simulink library "pathFollowingCtrlAoATurbCoef_cl"  (R2022a)
settings: Solver=VariableStepAuto  StartTime=0.0  StopTime=10.0  RelTol=1e-3
undefined symbols (not defined in the file or in its folder): env, FLIGHTCONTROLLER, initializeBussesFromBlock, pthCtrl1, vhcl
libraries: slpidlib x5, velocityAngle_ul x2, pathFollowingCtrlAoATurb_cl x1, courseFollowLookAhead_cl x1, ctrlAllocMatrix3CompCoef_cl x1, eulAng2RotMat_ul x1, angleBtw2Vecs_ul x1, vrlib x1, alphaBeta_ul x1, gnd2TanRotation_ul x1, rotorTorqueCtrlDiscrete x1
settings Model: Creator=jldanie5  LastModifiedBy=jbfine
settings SolverCC: AlgebraicLoopSolver=TrustRegion
settings DataIOCC: ReturnWorkspaceOutputs=off
settings DebuggingCC: UnconnectedInputMsg=warning  UnconnectedOutputMsg=warning  UnconnectedLineMsg=warning  SFMachineParentedDataDiag=warning  ArithmeticOperatorsInVariantConditions=warning
settings SFSimCC: CustomCodeUndefinedFunction=UseInterfaceOnly

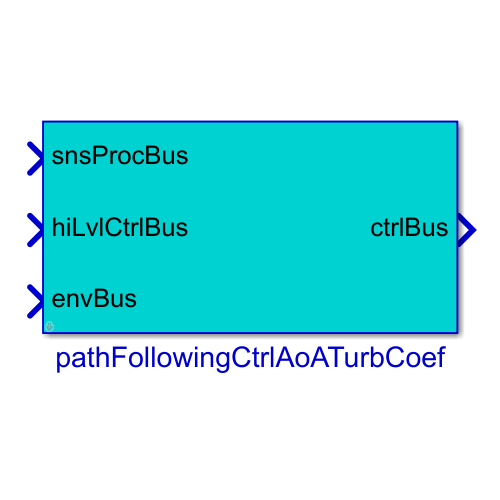
[thumbnail: Simulink's stored preview of the top-level diagram]
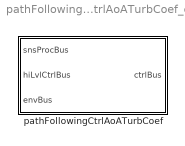
== system pathFollowingCtrlAoATurbCoef_cl ==
  pathFollowingCtrlAoATurbCoef : Subsystem  LoadFcn=initializeBussesFromBlock(gcb)  InitFcn=initializeBussesFromBlock(gcb)  StartFcn=initializeBussesFromBlock(gcb)  VariantControl=strcmpi(FLIGHTCONTROLLER,'pathFollowingControllerManta')  mask{initPosForInitSStar=vhcl.initPosVecGnd.Value, fluidDensity=env.water.density.Value, pathCtrl=pthCtrl1, aeroStruct=vhcl.struct('OCT.aeroSurf')}
      mask prompts: initPosForInitSStar "Initial Position"; fluidDensity "Fluid Density"; pathCtrl "Controller"; aeroStruct "Aerodynamic Structure"
      settings: MinAlgLoopOccurrences=on
      mask DialogControl Container3 Prompt: courseFollow Params
      mask DialogControl Container4 Prompt: setpointToOutput Params

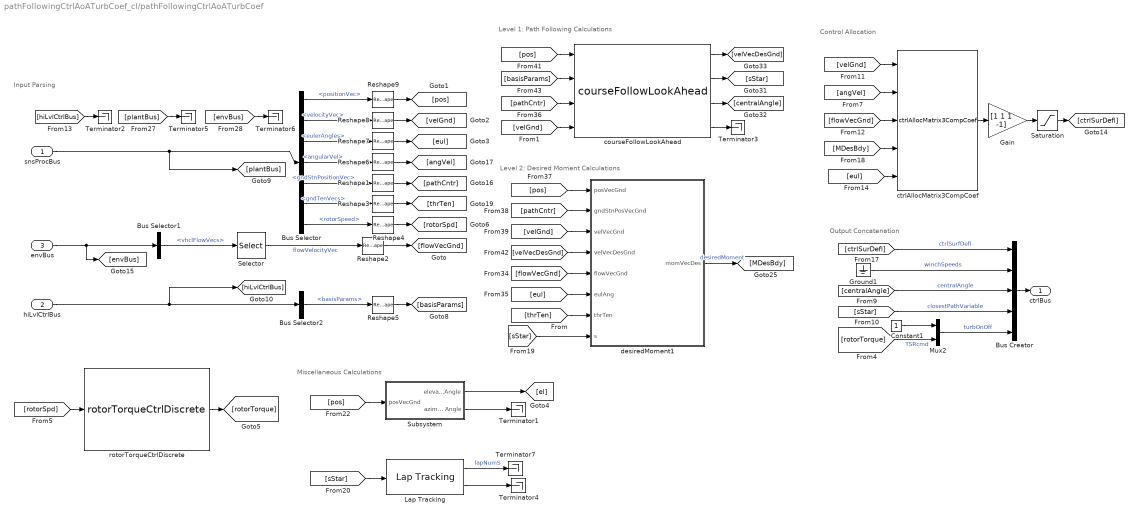
== system pathFollowingCtrlAoATurbCoef_cl/pathFollowingCtrlAoATurbCoef ==
  note: Control Allocation
  note: Miscellaneous Calculations
  note: Output Concatenation
  note: Input Parsing
  note: Level 1: Path Following Calculations
  note: Level 2: Desired Moment Calculations
  snsProcBus : Inport  OutDataTypeStr=Bus: sensorsProcessingBus
  hiLvlCtrlBus : Inport  Port=2
  envBus : Inport  Port=3  OutDataTypeStr=Bus: envBus
  Bus Creator : BusCreator  Inputs=5
  Bus Selector : BusSelector  OutputSignals=positionVec,velocityVec,eulerAngles,angularVel,gndStnPositionVec,gndTenVecs,rotorSpeed
  Bus Selector1 : BusSelector  OutputSignals=vhclFlowVecs
  Bus Selector2 : BusSelector  OutputSignals=basisParams
  Constant1 : Constant
  Gain : Gain  Gain=[1 1 1 -1]
  Ground1 : Ground
  Lap Tracking : pathFollowingCtrlAoATurb_cl/pathFollowingCtrlAoATurb/Lap Tracking  SystemSampleTime=-1  VariantActivationTime=update diagram  Latency=0  AutoFrameSizeCalculation=off
  Mux2 : Mux  Inputs=2
  Reshape{1..9} (9 alike) : Reshape  OutputDimensionality=Column vector (2-D)
  Saturation : Saturate  UpperLimit=30  LowerLimit=-30
  Selector : Selector  NumberOfDimensions=2  InputPortWidth=3  IndexOptions=Select all,Index vector (dialog)  Indices=[1 3],5  OutputSizes=1,1
  Subsystem : Subsystem
  Terminator{1..7} (7 alike) : Terminator
  courseFollowLookAhead : courseFollowLookAhead_cl/courseFollowLookAhead  SystemSampleTime=-1  VariantActivationTime=update diagram  Latency=0  AutoFrameSizeCalculation=off
  ctrlAllocMatrix3CompCoef : ctrlAllocMatrix3CompCoef_cl/ctrlAllocMatrix3CompCoef  aeroStruct=vhcl.struct('OCT.aeroSurf')  fluidDensity=fluidDensity  arms=vhcl.struct('OCT.thrAttch')
  desiredMoment1 : Subsystem
  rotorTorqueCtrlDiscrete : rotorTorqueCtrlDiscrete/rotorTorqueCtrlDiscrete  turb_struct=vhcl.struct('OCT.turb')  rho=rho
  ctrlBus : Outport  OutDataTypeStr=Bus: fltCtrlBus  VectorParamsAs1DForOutWhenUnconnected=off
  wires:
  Bus Selector/6 -> Reshape3/1  "<gndTenVecs>"
  Reshape3/1 -> [thrTen]
  snsProcBus/1 -> [plantBus], Bus Selector/1
  Bus Selector/2 -> Reshape8/1  "<velocityVec>"
  Bus Selector/1 -> Reshape9/1  "<positionVec>"
  Bus Selector/3 -> Reshape7/1  "<eulerAngles>"
  Bus Creator/1 -> ctrlBus/1
  Ground1/1 -> Bus Creator/2  "winchSpeeds"
  hiLvlCtrlBus/1 -> [hiLvlCtrlBus], Bus Selector2/1
  [centralAngle] -> Bus Creator/3  "centralAngle"
  [sStar] -> Bus Creator/4  "closestPathVariable"
  Bus Selector/4 -> Reshape6/1  "<angularVel>"
  [angVel] -> ctrlAllocMatrix3CompCoef/2
  [velGnd] -> ctrlAllocMatrix3CompCoef/1
  [flowVecGnd] -> ctrlAllocMatrix3CompCoef/3
  [MDesBdy] -> ctrlAllocMatrix3CompCoef/4
  [ctrlSurDefl] -> Bus Creator/1  "ctrlSurfDefl"
  Bus Selector2/1 -> Reshape5/1  "<basisParams>"
  Reshape5/1 -> [basisParams]
  Reshape2/1 -> [flowVecGnd]
  Reshape6/1 -> [angVel]
  Reshape7/1 -> [eul]
  Reshape8/1 -> [velGnd]
  Reshape9/1 -> [pos]
  [eul] -> ctrlAllocMatrix3CompCoef/5
  Selector/1 -> Reshape2/1  "flowVelocityVec"
  envBus/1 -> [envBus], Bus Selector1/1
  Bus Selector1/1 -> Selector/1  "<vhclFlowVecs>"
  Reshape1/1 -> [pathCntr]
  Bus Selector/5 -> Reshape1/1  "<gndStnPositionVec>"
  [pos] -> Subsystem/1(posVecGnd)
  Subsystem/2(azimuth Angle) -> Terminator1/1
  [plantBus] -> Terminator5/1
  [envBus] -> Terminator6/1
  [hiLvlCtrlBus] -> Terminator2/1
  Mux2/1 -> Bus Creator/5  "turbOnOff"
  Constant1/1 -> Mux2/1
  [rotorTorque] -> Mux2/2  "TSRcmd"
  [velVecDesGnd] -> desiredMoment1/4(velVecDesGnd)
  [velGnd] -> desiredMoment1/3(velVecGnd)
  [eul] -> desiredMoment1/6(eulAng)
  [basisParams] -> courseFollowLookAhead/2
  [pathCntr] -> desiredMoment1/2(gndStnPosVecGnd)
  courseFollowLookAhead/2 -> [sStar]
  [pos] -> desiredMoment1/1(posVecGnd)
  [pathCntr] -> courseFollowLookAhead/3
  desiredMoment1/1(momVecDes) -> [MDesBdy]  "desiredMoment"
  [pos] -> courseFollowLookAhead/1
  courseFollowLookAhead/3 -> [centralAngle]
  courseFollowLookAhead/4 -> Terminator3/1
  courseFollowLookAhead/1 -> [velVecDesGnd]
  [flowVecGnd] -> desiredMoment1/5(flowVecGnd)
  [thrTen] -> desiredMoment1/7(thrTen)
  [velGnd] -> courseFollowLookAhead/4
  Saturation/1 -> [ctrlSurDefl]
  [sStar] -> desiredMoment1/8(s)
  [rotorSpd] -> rotorTorqueCtrlDiscrete/1
  Reshape4/1 -> [rotorSpd]
  Bus Selector/7 -> Reshape4/1  "<rotorSpeed>"
  Subsystem/1(elevationAngle) -> [el]
  rotorTorqueCtrlDiscrete/1 -> [rotorTorque]
  ctrlAllocMatrix3CompCoef/1 -> Gain/1
  Gain/1 -> Saturation/1
  Lap Tracking/2 -> Terminator4/1
  Lap Tracking/1 -> Terminator7/1  "lapNumS"
  [sStar] -> Lap Tracking/1

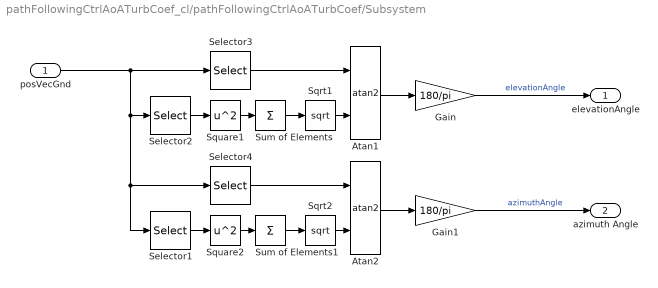
== system pathFollowingCtrlAoATurbCoef_cl/pathFollowingCtrlAoATurbCoef/Subsystem ==
  posVecGnd : Inport
  Atan1 : Trigonometry  Operator=atan2
  Atan2 : Trigonometry  Operator=atan2
  Gain : Gain  Gain=180/pi
  Gain1 : Gain  Gain=180/pi
  Selector1 : Selector  InputPortWidth=3  IndexOptions=Index vector (dialog)  Indices=1  OutputSizes=1
  Selector2 : Selector  InputPortWidth=3  IndexOptions=Index vector (dialog)  Indices=[1 2]  OutputSizes=1
  Selector3 : Selector  InputPortWidth=3  IndexOptions=Index vector (dialog)  Indices=3  OutputSizes=1
  Selector4 : Selector  InputPortWidth=3  IndexOptions=Index vector (dialog)  Indices=2  OutputSizes=1
  Sqrt1 : Sqrt
  Sqrt2 : Sqrt
  Square1 : Math  Operator=square  SignedPower=on
  Square2 : Math  Operator=square  SignedPower=on
  Sum of Elements : Sum  Inputs=+
  Sum of Elements1 : Sum  Inputs=+
  elevationAngle : Outport
  azimuth Angle : Outport  Port=2
  wires:
  Sqrt1/1 -> Atan1/2
  Square1/1 -> Sum of Elements/1
  Selector3/1 -> Atan1/1
  Sum of Elements/1 -> Sqrt1/1
  Atan1/1 -> Gain/1
  Selector2/1 -> Square1/1
  Gain/1 -> elevationAngle/1  "elevationAngle"
  Atan2/1 -> Gain1/1
  Square2/1 -> Sum of Elements1/1
  Sum of Elements1/1 -> Sqrt2/1
  Selector1/1 -> Square2/1
  posVecGnd/1 -> Selector1/1, Selector4/1, Selector2/1, Selector3/1
  Sqrt2/1 -> Atan2/2
  Selector4/1 -> Atan2/1
  Gain1/1 -> azimuth Angle/1  "azimuthAngle"

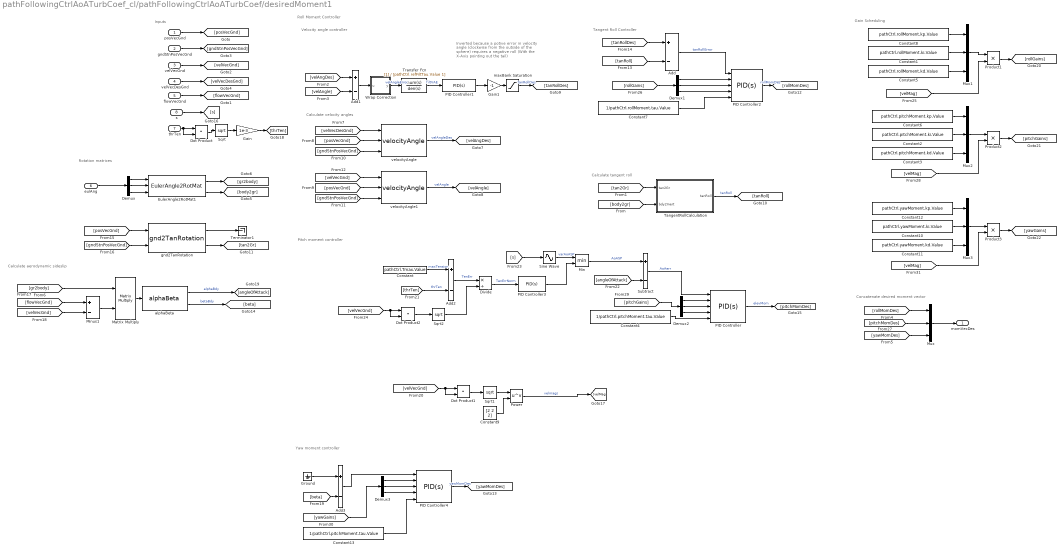
== system pathFollowingCtrlAoATurbCoef_cl/pathFollowingCtrlAoATurbCoef/desiredMoment1 ==
  note: Gain Scheduling
  note: Roll Moment Controller
  note: Calculate aerodynamic sideslip
  note: Concatenate desired moment vector
  note: Tangent Roll Controller
  note: Calculate tangent roll
  note: Calculate velocity angles
  note: Rotation matrices
  note: Inputs
  note: Velocity angle controller
  note: Inverted because a potive error
      | in velocity angle (clockwise from the
      | outside of the sphere) requires a negative
      | roll (With the X-Axis pointing out the tail)
  note: Pitch moment controller
  note: Yaw moment controller
  posVecGnd : Inport
  gndStnPosVecGnd : Inport  Port=2
  velVecGnd : Inport  Port=3
  velVecDesGnd : Inport  Port=4
  flowVecGnd : Inport  Port=5
  eulAng : Inport  Port=6
  thrTen : Inport  Port=7
  s : Inport  Port=8
  Add{,1..3} (4 alike) : Sum  Inputs=+-
  Constant : Constant  Value=pathCtrl.Tmax.Value
  Constant1 : Constant  Value=pathCtrl.rollMoment.ki.Value
  Constant10 : Constant  Value=pathCtrl.yawMoment.ki.Value
  Constant11 : Constant  Value=pathCtrl.yawMoment.kd.Value
  Constant12 : Constant  Value=pathCtrl.yawMoment.kp.Value
  Constant13 : Constant  Value=1/pathCtrl.pitchMoment.tau.Value
  Constant2 : Constant  Value=pathCtrl.pitchMoment.ki.Value
  Constant3 : Constant  Value=pathCtrl.pitchMoment.kd.Value
  Constant4 : Constant  Value=1/pathCtrl.pitchMoment.tau.Value
  Constant5 : Constant  Value=pathCtrl.rollMoment.kd.Value
  Constant6 : Constant  Value=pathCtrl.pitchMoment.kp.Value
  Constant7 : Constant  Value=1/pathCtrl.rollMoment.tau.Value
  Constant8 : Constant  Value=pathCtrl.rollMoment.kp.Value
  Constant9 : Constant  Value=[2 2 2]
  Demux{,1..3} (4 alike) : Demux  Outputs=3
  Divide : Product  Inputs=*/
  Dot Product : DotProduct  OutDataTypeStr=Inherit: Inherit via internal rule
  Dot Product1 : DotProduct  OutDataTypeStr=Inherit: Inherit via internal rule
  Dot Product2 : DotProduct  OutDataTypeStr=Inherit: Inherit via internal rule
  EulerAngle2RotMat1 : eulAng2RotMat_ul/EulerAngle2RotMat  SystemSampleTime=-1  VariantActivationTime=update diagram  Latency=0  AutoFrameSizeCalculation=off
  Gain : Gain  Gain=1e-3
  Gain1 : Gain  Gain=-1
  Ground : Ground
  Matrix Multiply : Product  Multiplication=Matrix(*)
  Min : MinMax  Inputs=2
  Minus1 : Sum  Inputs=+-
  Mux{,1..3} (4 alike) : Mux  Inputs=3
  PID Controller : slpidlib/PID Controller  Controller=PID  Form=Parallel  TimeDomain=Continuous-time  UseExternalTs=off  SampleTime=-1  IntegratorMethod=Forward Euler  FilterMethod=Forward Euler  ControllerParametersSource=external  P=pathCtrl.pitchMoment.kp.Value  I=pathCtrl.pitchMoment.ki.Value  UseKiTs=off  D=pathCtrl.pitchMoment.kd.Value  N=1/pathCtrl.pitchMoment.tau.Value  UseFilter=on  TunerSelectOption=Transfer Function Based (PID Tuner App)  InitialConditionSource=internal  InitialConditionForIntegrator=0  InitialConditionForFilter=0  DifferentiatorICPrevScaledInput=0  ExternalReset=none  TrackingMode=off  Kt=1  LimitOutput=off  SatLimitsSource=internal  UpperSaturationLimit=inf  LowerSaturationLimit=-100  LinearizeAsGain=on  AntiWindupMode=clamping  Kb=1  POutMin=[]  POutMax=[]  IOutMin=[]  IOutMax=[]  DOutMin=[]  DOutMax=[]  NOutMin=[]  NOutMax=[]  SumOutMin=[]  SumOutMax=[]  SaturationOutMin=[]  SaturationOutMax=[]  PParamMin=[]  PParamMax=[]  IParamMin=[]  IParamMax=[]  DParamMin=[]  DParamMax=[]  NParamMin=[]  NParamMax=[]  KbParamMin=[]  KbParamMax=[]  KtParamMin=[]  KtParamMax=[]  KbOutMin=[]  KbOutMax=[]  KtOutMin=[]  KtOutMax=[]  IntegratorOutMin=[]  IntegratorOutMax=[]  FilterOutMin=[]  FilterOutMax=[]  SumI1OutMin=[]  SumI1OutMax=[]  SumI2OutMin=[]  SumI2OutMax=[]  SumI3OutMin=[]  SumI3OutMax=[]  SumI4OutMin=[]  SumI4OutMax=[]  SumDOutMin=[]  SumDOutMax=[]  DifferentiatorOutMin=[]  DifferentiatorOutMax=[]  FilterDiffOutCoefMin=[]  FilterDiffOutCoefMax=[]  ReciprocalOutMin=[]  ReciprocalOutMax=[]  SumDenOutMin=[]  SumDenOutMax=[]  SumNumOutMin=[]  SumNumOutMax=[]  DivideOutMin=[]  DivideOutMax=[]  UdiffTsProdOutMin=[]  UdiffTsProdOutMax=[]  NTsProdOutMin=[]  NTsProdOutMax=[]  UintegralTsProdOutMin=[]  UintegralTsProdOutMax=[]  UngainTsProdOutMin=[]  UngainTsProdOutMax=[]  IntegratorContinuousStateAttributes=''  IntegratorStateMustResolveToSignalObject=off  IntegratorRTWStateStorageClass=Auto  FilterContinuousStateAttributes=''  FilterStateMustResolveToSignalObject=off  FilterRTWStateStorageClass=Auto  ParallelPVariant=ExternalParameters  IdealPVariant=Disabled  IVariant=ExternalParameters  DVariant=ExternalParameters  IntegratorVariant=Continuous  SatVariant=Disabled  AWVariant=Passthrough  PCopyVariant=Disabled  TRVariant=Disabled  FdbkBlocksVariant=Forward  IdealPFdbkVariant=Disabled  SatFdbkVariant=Disabled  DerivativeFilterVariant=ContFilter  NVariant=ExternalParameters  NCopyVariant=Disabled  FilterICVariant=InternalICsFilter  IntegratorICVariant=InternalICs  ExternalResetVariant=Disabled  TRSumVariant=Passthrough  SumFdbkVariant=Disabled  SumVariant=Sum_PID  TsampFilterVariant=InternalTs  TsampNgainVariant=Passthrough  TsampIntegralVariant=Passthrough  ExternalSaturationOutDataTypeStr=Inherit: Same as second input  aMode=0
  PID Controller1 : slpidlib/PID Controller  Controller=PID  Form=Parallel  TimeDomain=Continuous-time  UseExternalTs=off  SampleTime=-1  IntegratorMethod=Forward Euler  FilterMethod=Forward Euler  ControllerParametersSource=internal  P=pathCtrl.tanRoll.kp.Value  I=pathCtrl.tanRoll.ki.Value  UseKiTs=off  D=pathCtrl.tanRoll.kd.Value  N=1/pathCtrl.tanRoll.tau.Value  UseFilter=on  TunerSelectOption=Transfer Function Based (PID Tuner App)  InitialConditionSource=internal  InitialConditionForIntegrator=0  InitialConditionForFilter=0  DifferentiatorICPrevScaledInput=0  ExternalReset=none  TrackingMode=off  Kt=1  LimitOutput=off  SatLimitsSource=internal  UpperSaturationLimit=inf  LowerSaturationLimit=-100  LinearizeAsGain=on  AntiWindupMode=clamping  Kb=1  POutMin=[]  POutMax=[]  IOutMin=[]  IOutMax=[]  DOutMin=[]  DOutMax=[]  NOutMin=[]  NOutMax=[]  SumOutMin=[]  SumOutMax=[]  SaturationOutMin=[]  SaturationOutMax=[]  PParamMin=[]  PParamMax=[]  IParamMin=[]  IParamMax=[]  DParamMin=[]  DParamMax=[]  NParamMin=[]  NParamMax=[]  KbParamMin=[]  KbParamMax=[]  KtParamMin=[]  KtParamMax=[]  KbOutMin=[]  KbOutMax=[]  KtOutMin=[]  KtOutMax=[]  IntegratorOutMin=[]  IntegratorOutMax=[]  FilterOutMin=[]  FilterOutMax=[]  SumI1OutMin=[]  SumI1OutMax=[]  SumI2OutMin=[]  SumI2OutMax=[]  SumI3OutMin=[]  SumI3OutMax=[]  SumI4OutMin=[]  SumI4OutMax=[]  SumDOutMin=[]  SumDOutMax=[]  DifferentiatorOutMin=[]  DifferentiatorOutMax=[]  FilterDiffOutCoefMin=[]  FilterDiffOutCoefMax=[]  ReciprocalOutMin=[]  ReciprocalOutMax=[]  SumDenOutMin=[]  SumDenOutMax=[]  SumNumOutMin=[]  SumNumOutMax=[]  DivideOutMin=[]  DivideOutMax=[]  UdiffTsProdOutMin=[]  UdiffTsProdOutMax=[]  NTsProdOutMin=[]  NTsProdOutMax=[]  UintegralTsProdOutMin=[]  UintegralTsProdOutMax=[]  UngainTsProdOutMin=[]  UngainTsProdOutMax=[]  IntegratorContinuousStateAttributes=''  IntegratorStateMustResolveToSignalObject=off  IntegratorRTWStateStorageClass=Auto  FilterContinuousStateAttributes=''  FilterStateMustResolveToSignalObject=off  FilterRTWStateStorageClass=Auto  ParallelPVariant=InternalParameters  IdealPVariant=Disabled  IVariant=InternalParameters  DVariant=InternalParameters  IntegratorVariant=Continuous  SatVariant=Disabled  AWVariant=Passthrough  PCopyVariant=Disabled  TRVariant=Disabled  FdbkBlocksVariant=Forward  IdealPFdbkVariant=Disabled  SatFdbkVariant=Disabled  DerivativeFilterVariant=ContFilter  NVariant=InternalParameters  NCopyVariant=Disabled  FilterICVariant=InternalICsFilter  IntegratorICVariant=InternalICs  ExternalResetVariant=Disabled  TRSumVariant=Passthrough  SumFdbkVariant=Disabled  SumVariant=Sum_PID  TsampFilterVariant=InternalTs  TsampNgainVariant=Passthrough  TsampIntegralVariant=Passthrough  ExternalSaturationOutDataTypeStr=Inherit: Same as second input  aMode=0
  PID Controller2 : slpidlib/PID Controller  Controller=PID  Form=Parallel  TimeDomain=Continuous-time  UseExternalTs=off  SampleTime=-1  IntegratorMethod=Forward Euler  FilterMethod=Forward Euler  ControllerParametersSource=external  P=pathCtrl.rollMoment.kp.Value  I=pathCtrl.rollMoment.ki.Value  UseKiTs=off  D=pathCtrl.rollMoment.kd.Value  N=1/pathCtrl.rollMoment.tau.Value  UseFilter=on  TunerSelectOption=Transfer Function Based (PID Tuner App)  InitialConditionSource=internal  InitialConditionForIntegrator=0  InitialConditionForFilter=0  DifferentiatorICPrevScaledInput=0  ExternalReset=none  TrackingMode=off  Kt=1  LimitOutput=off  SatLimitsSource=internal  UpperSaturationLimit=inf  LowerSaturationLimit=-100  LinearizeAsGain=on  AntiWindupMode=clamping  Kb=1  POutMin=[]  POutMax=[]  IOutMin=[]  IOutMax=[]  DOutMin=[]  DOutMax=[]  NOutMin=[]  NOutMax=[]  SumOutMin=[]  SumOutMax=[]  SaturationOutMin=[]  SaturationOutMax=[]  PParamMin=[]  PParamMax=[]  IParamMin=[]  IParamMax=[]  DParamMin=[]  DParamMax=[]  NParamMin=[]  NParamMax=[]  KbParamMin=[]  KbParamMax=[]  KtParamMin=[]  KtParamMax=[]  KbOutMin=[]  KbOutMax=[]  KtOutMin=[]  KtOutMax=[]  IntegratorOutMin=[]  IntegratorOutMax=[]  FilterOutMin=[]  FilterOutMax=[]  SumI1OutMin=[]  SumI1OutMax=[]  SumI2OutMin=[]  SumI2OutMax=[]  SumI3OutMin=[]  SumI3OutMax=[]  SumI4OutMin=[]  SumI4OutMax=[]  SumDOutMin=[]  SumDOutMax=[]  DifferentiatorOutMin=[]  DifferentiatorOutMax=[]  FilterDiffOutCoefMin=[]  FilterDiffOutCoefMax=[]  ReciprocalOutMin=[]  ReciprocalOutMax=[]  SumDenOutMin=[]  SumDenOutMax=[]  SumNumOutMin=[]  SumNumOutMax=[]  DivideOutMin=[]  DivideOutMax=[]  UdiffTsProdOutMin=[]  UdiffTsProdOutMax=[]  NTsProdOutMin=[]  NTsProdOutMax=[]  UintegralTsProdOutMin=[]  UintegralTsProdOutMax=[]  UngainTsProdOutMin=[]  UngainTsProdOutMax=[]  IntegratorContinuousStateAttributes=''  IntegratorStateMustResolveToSignalObject=off  IntegratorRTWStateStorageClass=Auto  FilterContinuousStateAttributes=''  FilterStateMustResolveToSignalObject=off  FilterRTWStateStorageClass=Auto  ParallelPVariant=ExternalParameters  IdealPVariant=Disabled  IVariant=ExternalParameters  DVariant=ExternalParameters  IntegratorVariant=Continuous  SatVariant=Disabled  AWVariant=Passthrough  PCopyVariant=Disabled  TRVariant=Disabled  FdbkBlocksVariant=Forward  IdealPFdbkVariant=Disabled  SatFdbkVariant=Disabled  DerivativeFilterVariant=ContFilter  NVariant=ExternalParameters  NCopyVariant=Disabled  FilterICVariant=InternalICsFilter  IntegratorICVariant=InternalICs  ExternalResetVariant=Disabled  TRSumVariant=Passthrough  SumFdbkVariant=Disabled  SumVariant=Sum_PID  TsampFilterVariant=InternalTs  TsampNgainVariant=Passthrough  TsampIntegralVariant=Passthrough  ExternalSaturationOutDataTypeStr=Inherit: Same as second input  aMode=0
  PID Controller3 : slpidlib/PID Controller  Controller=PID  Form=Parallel  TimeDomain=Continuous-time  UseExternalTs=off  SampleTime=-1  IntegratorMethod=Forward Euler  FilterMethod=Forward Euler  ControllerParametersSource=internal  P=pathCtrl.alphaCtrl.kp.Value  I=pathCtrl.alphaCtrl.ki.Value  UseKiTs=off  D=pathCtrl.alphaCtrl.kd.Value  N=1/pathCtrl.alphaCtrl.tau.Value  UseFilter=on  TunerSelectOption=Transfer Function Based (PID Tuner App)  InitialConditionSource=internal  InitialConditionForIntegrator=0  InitialConditionForFilter=0  DifferentiatorICPrevScaledInput=0  ExternalReset=none  TrackingMode=off  Kt=1  LimitOutput=on  SatLimitsSource=internal  UpperSaturationLimit=pathCtrl.AoAConst.Value  LowerSaturationLimit=pathCtrl.AoAmin.Value  LinearizeAsGain=on  AntiWindupMode=clamping  Kb=1  POutMin=[]  POutMax=[]  IOutMin=[]  IOutMax=[]  DOutMin=[]  DOutMax=[]  NOutMin=[]  NOutMax=[]  SumOutMin=[]  SumOutMax=[]  SaturationOutMin=[]  SaturationOutMax=[]  PParamMin=[]  PParamMax=[]  IParamMin=[]  IParamMax=[]  DParamMin=[]  DParamMax=[]  NParamMin=[]  NParamMax=[]  KbParamMin=[]  KbParamMax=[]  KtParamMin=[]  KtParamMax=[]  KbOutMin=[]  KbOutMax=[]  KtOutMin=[]  KtOutMax=[]  IntegratorOutMin=[]  IntegratorOutMax=[]  FilterOutMin=[]  FilterOutMax=[]  SumI1OutMin=[]  SumI1OutMax=[]  SumI2OutMin=[]  SumI2OutMax=[]  SumI3OutMin=[]  SumI3OutMax=[]  SumI4OutMin=[]  SumI4OutMax=[]  SumDOutMin=[]  SumDOutMax=[]  DifferentiatorOutMin=[]  DifferentiatorOutMax=[]  FilterDiffOutCoefMin=[]  FilterDiffOutCoefMax=[]  ReciprocalOutMin=[]  ReciprocalOutMax=[]  SumDenOutMin=[]  SumDenOutMax=[]  SumNumOutMin=[]  SumNumOutMax=[]  DivideOutMin=[]  DivideOutMax=[]  UdiffTsProdOutMin=[]  UdiffTsProdOutMax=[]  NTsProdOutMin=[]  NTsProdOutMax=[]  UintegralTsProdOutMin=[]  UintegralTsProdOutMax=[]  UngainTsProdOutMin=[]  UngainTsProdOutMax=[]  IntegratorContinuousStateAttributes=''  IntegratorStateMustResolveToSignalObject=off  IntegratorRTWStateStorageClass=Auto  FilterContinuousStateAttributes=''  FilterStateMustResolveToSignalObject=off  FilterRTWStateStorageClass=Auto  ParallelPVariant=InternalParameters  IdealPVariant=Disabled  IVariant=InternalParameters  DVariant=InternalParameters  IntegratorVariant=Continuous  SatVariant=Enabled  AWVariant=ContClampingParallel  PCopyVariant=Disabled  TRVariant=Disabled  FdbkBlocksVariant=Forward  IdealPFdbkVariant=Disabled  SatFdbkVariant=Disabled  DerivativeFilterVariant=ContFilter  NVariant=InternalParameters  NCopyVariant=Disabled  FilterICVariant=InternalICsFilter  IntegratorICVariant=InternalICs  ExternalResetVariant=Disabled  TRSumVariant=Passthrough  SumFdbkVariant=Disabled  SumVariant=Sum_PID  TsampFilterVariant=InternalTs  TsampNgainVariant=Passthrough  TsampIntegralVariant=Passthrough  ExternalSaturationOutDataTypeStr=Inherit: Same as second input  aMode=0
  PID Controller4 : slpidlib/PID Controller  Controller=PID  Form=Parallel  TimeDomain=Continuous-time  UseExternalTs=off  SampleTime=-1  IntegratorMethod=Forward Euler  FilterMethod=Forward Euler  ControllerParametersSource=external  P=pathCtrl.pitchMoment.kp.Value  I=pathCtrl.pitchMoment.ki.Value  UseKiTs=off  D=pathCtrl.pitchMoment.kd.Value  N=1/pathCtrl.pitchMoment.tau.Value  UseFilter=on  TunerSelectOption=Transfer Function Based (PID Tuner App)  InitialConditionSource=internal  InitialConditionForIntegrator=0  InitialConditionForFilter=0  DifferentiatorICPrevScaledInput=0  ExternalReset=none  TrackingMode=off  Kt=1  LimitOutput=off  SatLimitsSource=internal  UpperSaturationLimit=inf  LowerSaturationLimit=-100  LinearizeAsGain=on  AntiWindupMode=clamping  Kb=1  POutMin=[]  POutMax=[]  IOutMin=[]  IOutMax=[]  DOutMin=[]  DOutMax=[]  NOutMin=[]  NOutMax=[]  SumOutMin=[]  SumOutMax=[]  SaturationOutMin=[]  SaturationOutMax=[]  PParamMin=[]  PParamMax=[]  IParamMin=[]  IParamMax=[]  DParamMin=[]  DParamMax=[]  NParamMin=[]  NParamMax=[]  KbParamMin=[]  KbParamMax=[]  KtParamMin=[]  KtParamMax=[]  KbOutMin=[]  KbOutMax=[]  KtOutMin=[]  KtOutMax=[]  IntegratorOutMin=[]  IntegratorOutMax=[]  FilterOutMin=[]  FilterOutMax=[]  SumI1OutMin=[]  SumI1OutMax=[]  SumI2OutMin=[]  SumI2OutMax=[]  SumI3OutMin=[]  SumI3OutMax=[]  SumI4OutMin=[]  SumI4OutMax=[]  SumDOutMin=[]  SumDOutMax=[]  DifferentiatorOutMin=[]  DifferentiatorOutMax=[]  FilterDiffOutCoefMin=[]  FilterDiffOutCoefMax=[]  ReciprocalOutMin=[]  ReciprocalOutMax=[]  SumDenOutMin=[]  SumDenOutMax=[]  SumNumOutMin=[]  SumNumOutMax=[]  DivideOutMin=[]  DivideOutMax=[]  UdiffTsProdOutMin=[]  UdiffTsProdOutMax=[]  NTsProdOutMin=[]  NTsProdOutMax=[]  UintegralTsProdOutMin=[]  UintegralTsProdOutMax=[]  UngainTsProdOutMin=[]  UngainTsProdOutMax=[]  IntegratorContinuousStateAttributes=''  IntegratorStateMustResolveToSignalObject=off  IntegratorRTWStateStorageClass=Auto  FilterContinuousStateAttributes=''  FilterStateMustResolveToSignalObject=off  FilterRTWStateStorageClass=Auto  ParallelPVariant=ExternalParameters  IdealPVariant=Disabled  IVariant=ExternalParameters  DVariant=ExternalParameters  IntegratorVariant=Continuous  SatVariant=Disabled  AWVariant=Passthrough  PCopyVariant=Disabled  TRVariant=Disabled  FdbkBlocksVariant=Forward  IdealPFdbkVariant=Disabled  SatFdbkVariant=Disabled  DerivativeFilterVariant=ContFilter  NVariant=ExternalParameters  NCopyVariant=Disabled  FilterICVariant=InternalICsFilter  IntegratorICVariant=InternalICs  ExternalResetVariant=Disabled  TRSumVariant=Passthrough  SumFdbkVariant=Disabled  SumVariant=Sum_PID  TsampFilterVariant=InternalTs  TsampNgainVariant=Passthrough  TsampIntegralVariant=Passthrough  ExternalSaturationOutDataTypeStr=Inherit: Same as second input  aMode=0
  Power : Math  Operator=pow
  Product1 : Product
  Product2 : Product
  Product3 : Product
  Sine Wave : Sin  TimeSource=Use external signal  Amplitude=2*pi/180  Bias=13*pi/180  Frequency=4*pi  Phase=pi/2  SampleTime=0
  Sqrt : Sqrt
  Sqrt1 : Sqrt
  Sqrt2 : Sqrt
  Subtract : Sum  Inputs=+-
  TangentRollCalculation : Subsystem
  Terminator1 : Terminator
  Transfer Fcn : TransferFcn  Denominator=[pathCtrl.refFiltTau.Value 1]
  Wrap Correction : Subsystem
  alphaBeta : alphaBeta_ul/alphaBeta  SystemSampleTime=-1  VariantActivationTime=update diagram  Latency=0  AutoFrameSizeCalculation=off
  gnd2TanRotation : gnd2TanRotation_ul/gnd2TanRotation  SystemSampleTime=-1  VariantActivationTime=update diagram  Latency=0  AutoFrameSizeCalculation=off
  maxBank Saturation : Saturate  UpperLimit=pathCtrl.maxBank.upperLimit.Value  LowerLimit=pathCtrl.maxBank.lowerLimit.Value
  velocityAngle : velocityAngle_ul/velocityAngle  SystemSampleTime=-1  VariantActivationTime=update diagram  Latency=0  AutoFrameSizeCalculation=off
  velocityAngle1 : velocityAngle_ul/velocityAngle  SystemSampleTime=-1  VariantActivationTime=update diagram  Latency=0  AutoFrameSizeCalculation=off
  momVecDes : Outport  VectorParamsAs1DForOutWhenUnconnected=off
  wires:
  PID Controller2/1 -> [rollMomDes]  "rollMomDes"
  [rollMomDes] -> Mux/1
  Wrap Correction/1(y) -> Transfer Fcn/1  "velAngleError"
  posVecGnd/1 -> [posVecGnd]
  velVecGnd/1 -> [velVecGnd]
  Add/1 -> PID Controller2/1  "tanRollError"
  Gain1/1 -> maxBank Saturation/1
  maxBank Saturation/1 -> [tanRollDes]  "tanRollDes"
  Add1/1 -> Wrap Correction/1(u)
  flowVecGnd/1 -> [flowVecGnd]
  [tan2Gr] -> TangentRollCalculation/1(tan2Gr)
  TangentRollCalculation/1(tanRoll) -> [tanRoll]  "tanRoll"
  Minus1/1 -> Matrix Multiply/2
  [velVecGnd] -> Minus1/2
  [flowVecGnd] -> Minus1/1
  eulAng/1 -> Demux/1
  Demux/2 -> EulerAngle2RotMat1/2
  EulerAngle2RotMat1/2 -> [body2gr]
  EulerAngle2RotMat1/1 -> [gr2body]
  [body2gr] -> TangentRollCalculation/2(bdy2Inert)
  [gr2body] -> Matrix Multiply/1
  Matrix Multiply/1 -> alphaBeta/1
  alphaBeta/2 -> [beta]  "betaBdy"
  alphaBeta/1 -> [angleOfAttack]  "alphaBdy"
  gndStnPosVecGnd/1 -> [gndStnPosVecGnd]
  velVecDesGnd/1 -> [velVecDesGnd]
  velocityAngle/1 -> [velAngDes]  "velAngleDes"
  velocityAngle1/1 -> [velAngle]  "velAngle"
  [velAngDes] -> Add1/1
  [velAngle] -> Add1/2
  [velVecDesGnd] -> velocityAngle/1
  [posVecGnd] -> velocityAngle/2
  [posVecGnd] -> velocityAngle1/2
  [gndStnPosVecGnd] -> velocityAngle/3
  [gndStnPosVecGnd] -> velocityAngle1/3
  [velVecGnd] -> velocityAngle1/1
  [tanRoll] -> Add/2
  [tanRollDes] -> Add/1
  [posVecGnd] -> gnd2TanRotation/1
  [gndStnPosVecGnd] -> gnd2TanRotation/2
  gnd2TanRotation/2 -> [tan2Gr]
  gnd2TanRotation/1 -> Terminator1/1
  [yawMomDes] -> Mux/3
  PID Controller1/1 -> Gain1/1
  [beta] -> Add3/2
  Ground/1 -> Add3/1
  [pitchMomDes] -> Mux/2
  PID Controller4/1 -> [yawMomDes]  "yawMomDes"
  PID Controller/1 -> [pitchMomDes]  "elevMom"
  [angleOfAttack] -> Subtract/2
  Subtract/1 -> PID Controller/1  "AoAerr"
  thrTen/1 -> Dot Product/2, Dot Product/1
  Sqrt/1 -> Gain/1
  Dot Product/1 -> Sqrt/1
  Gain/1 -> [thrTen]
  Demux/1 -> EulerAngle2RotMat1/1
  Demux/3 -> EulerAngle2RotMat1/3
  Mux/1 -> momVecDes/1
  Transfer Fcn/1 -> PID Controller1/1  "filtVAE"
  [thrTen] -> Add2/2  "thrTen"
  Add2/1 -> Divide/1  "TenErr"
  Constant/1 -> Add2/1  "maxTension"
  Divide/1 -> PID Controller3/1  "TenErrNorm"
  Constant4/1 -> PID Controller/5
  s/1 -> [s]
  [s] -> Sine Wave/1
  Sine Wave/1 -> Min/1  "varAoASP"
  PID Controller3/1 -> Min/2
  Demux1/3 -> PID Controller2/4
  Demux1/1 -> PID Controller2/2
  Constant7/1 -> PID Controller2/5
  Demux1/2 -> PID Controller2/3
  Dot Product1/1 -> Sqrt1/1
  [velVecGnd] -> Dot Product1/2, Dot Product1/1
  Constant5/1 -> Mux1/3
  Constant1/1 -> Mux1/2
  Constant8/1 -> Mux1/1
  Mux1/1 -> Product1/1
  [velMag] -> Product1/2
  Product1/1 -> [rollGains]
  [rollGains] -> Demux1/1
  Mux2/1 -> Product2/1
  Constant6/1 -> Mux2/1
  Constant2/1 -> Mux2/2
  Constant3/1 -> Mux2/3
  Product2/1 -> [pitchGains]
  [velMag] -> Product2/2
  Demux2/2 -> PID Controller/3
  Demux2/1 -> PID Controller/2
  [pitchGains] -> Demux2/1
  Demux2/3 -> PID Controller/4
  Min/1 -> Subtract/1  "AoASP"
  Sqrt1/1 -> Power/1
  Constant9/1 -> Power/2
  Power/1 -> [velMag]  "velmags"
  Dot Product2/1 -> Sqrt2/1
  [velVecGnd] -> Dot Product2/2, Dot Product2/1
  Sqrt2/1 -> Divide/2
  [velMag] -> Product3/2
  Product3/1 -> [yawGains]
  Mux3/1 -> Product3/1
  Constant10/1 -> Mux3/2
  Constant11/1 -> Mux3/3
  Constant12/1 -> Mux3/1
  Demux3/2 -> PID Controller4/3
  [yawGains] -> Demux3/1
  Demux3/3 -> PID Controller4/4
  Constant13/1 -> PID Controller4/5
  Demux3/1 -> PID Controller4/2
  Add3/1 -> PID Controller4/1

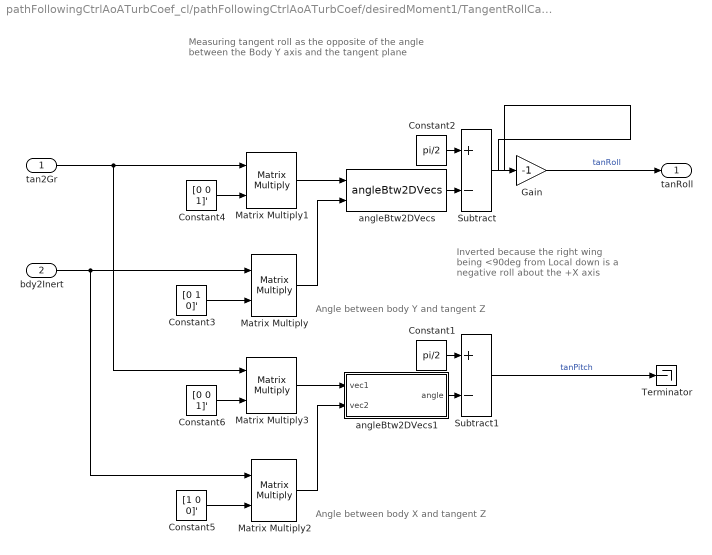
== system pathFollowingCtrlAoATurbCoef_cl/pathFollowingCtrlAoATurbCoef/desiredMoment1/TangentRollCalculation ==
  note: Measuring tangent roll as the opposite
      | of the angle between the Body Y axis
      | and the tangent plane
  note: Angle between body Y and tangent Z
  note: Inverted because the right wing
      | being <90deg from Local down
      | is a negative roll about the +X axis
  note: Angle between body X and tangent Z
  tan2Gr : Inport
  bdy2Inert : Inport  Port=2
  Constant1 : Constant  Value=pi/2
  Constant2 : Constant  Value=pi/2
  Constant3 : Constant  Value=[0 1 0]'
  Constant4 : Constant  Value=[0 0 1]'
  Constant5 : Constant  Value=[1 0 0]'
  Constant6 : Constant  Value=[0 0 1]'
  Gain : Gain  Gain=-1
  Matrix Multiply{,1..3} (4 alike) : Product  Multiplication=Matrix(*)
  Subtract : Sum  Inputs=+-
  Subtract1 : Sum  Inputs=+-
  Terminator : Terminator
  angleBtw2DVecs : angleBtw2Vecs_ul/angleBtw2DVecs  SystemSampleTime=-1  VariantActivationTime=update diagram  Latency=0  AutoFrameSizeCalculation=off
  angleBtw2DVecs1 : Subsystem
  tanRoll : Outport  VectorParamsAs1DForOutWhenUnconnected=off
  wires:
  Subtract/1 -> Gain/1
  Constant3/1 -> Matrix Multiply/2
  angleBtw2DVecs/1 -> Subtract/2
  Constant2/1 -> Subtract/1
  Matrix Multiply1/1 -> angleBtw2DVecs/1
  Constant4/1 -> Matrix Multiply1/2
  Matrix Multiply/1 -> angleBtw2DVecs/2
  Gain/1 -> tanRoll/1  "tanRoll"
  bdy2Inert/1 -> Matrix Multiply2/1, Matrix Multiply/1
  Subtract1/1 -> Terminator/1  "tanPitch"
  tan2Gr/1 -> Matrix Multiply3/1, Matrix Multiply1/1
  Matrix Multiply2/1 -> angleBtw2DVecs1/2(vec2)
  Constant6/1 -> Matrix Multiply3/2
  Matrix Multiply3/1 -> angleBtw2DVecs1/1(vec1)
  Constant1/1 -> Subtract1/1
  angleBtw2DVecs1/1(angle) -> Subtract1/2
  Constant5/1 -> Matrix Multiply2/2

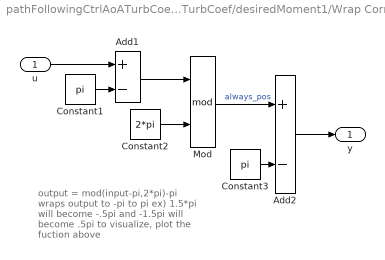
== system pathFollowingCtrlAoATurbCoef_cl/pathFollowingCtrlAoATurbCoef/desiredMoment1/Wrap Correction ==
  note: output = mod(input-pi,2*pi)-pi
      | wraps output to -pi to pi
      |
      | ex) 1.5*pi will become -.5pi
      | 	and -1.5pi will become .5pi
      |
      | to visualize, plot the fuction above
  u : Inport
  Add1 : Sum  Inputs=+-
  Add2 : Sum  Inputs=+-
  Constant1 : Constant  Value=pi
  Constant2 : Constant  Value=2*pi
  Constant3 : Constant  Value=pi
  Mod : Math  Operator=mod  SignedPower=on
  y : Outport  VectorParamsAs1DForOutWhenUnconnected=off
  wires:
  u/1 -> Add1/1
  Constant1/1 -> Add1/2
  Add1/1 -> Mod/1
  Constant2/1 -> Mod/2
  Mod/1 -> Add2/1  "always_pos"
  Constant3/1 -> Add2/2
  Add2/1 -> y/1

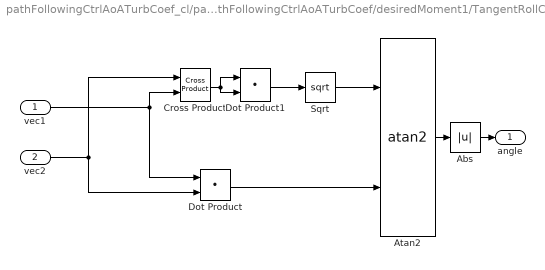
== system pathFollowingCtrlAoATurbCoef_cl/pathFollowingCtrlAoATurbCoef/desiredMoment1/TangentRollCalculation/angleBtw2DVecs1 ==
  vec1 : Inport
  vec2 : Inport  Port=2
  Abs : Abs  SaturateOnIntegerOverflow=off
  Atan2 : Trigonometry  Operator=atan2
  Cross Product : vrlib/Utilities/Cross Product
  Dot Product : DotProduct  OutDataTypeStr=Inherit: Inherit via internal rule
  Dot Product1 : DotProduct  OutDataTypeStr=Inherit: Inherit via internal rule
  Sqrt : Sqrt
  angle : Outport  VectorParamsAs1DForOutWhenUnconnected=off
  wires:
  Atan2/1 -> Abs/1
  vec1/1 -> Dot Product/1, Cross Product/2
  vec2/1 -> Cross Product/1, Dot Product/2
  Cross Product/1 -> Dot Product1/1, Dot Product1/2
  Dot Product/1 -> Atan2/2
  Abs/1 -> angle/1
  Dot Product1/1 -> Sqrt/1
  Sqrt/1 -> Atan2/1
